simulink model "controller_for_carsim"  (R2021a)
settings: Solver=VariableStepAuto  StartTime=0.0  StopTime=10  RelTol=1e-2
undefined symbols (not defined in the file): Fyf, ks, PredictionHorizon, SlipAngle, Ts, Vx
libraries: mpclib x1, Solver_SF x1, simulink_extras x1, simulink x1
settings Model: Creator=dekunw  LastModifiedBy=chnwa
settings SolverCC: AlgebraicLoopSolver=LineSearch
settings DebuggingCC: SFMachineParentedDataDiag=warning

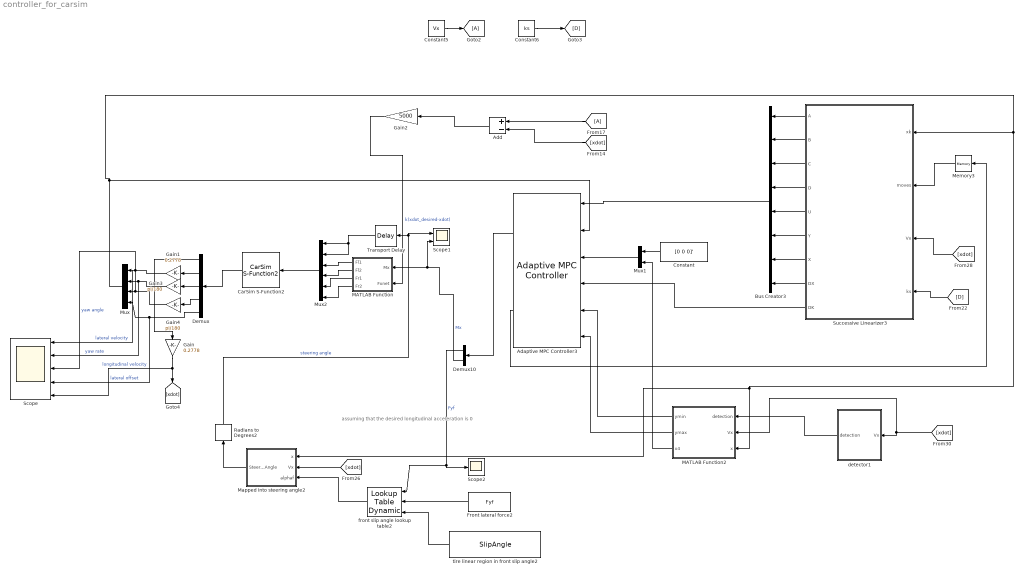
== system controller_for_carsim ==
  note: assuming that the desired longitudinal acceleration is 0
  Adaptive MPC Controller3 : mpclib/Adaptive MPC Controller  SCDEnableBlockLinearizationSpecification=on  mpcobj=mpc007  enable_value=0  updateMPCinCallerWorkspace=on  md_inport=on  mv_inport=off  uref_inport=off  return_cost=off  return_mvseq=on  return_qpstatus=off  return_xseq=off  return_state=off  return_ovseq=off  state_inport=off  isltv_plant=on  umin_inport=off  umax_inport=off  ymin_inport=on  ymax_inport=on  cc_inport=off  ywt_inport=off  uwt_inport=off  duwt_inport=off  rhoeps_inport=off  pm_inport=off  MaximumP=10  HorizonChoice=FixedHorizon  BlockDataType=double  SampleTimeInherited=off  switch_inport=off
  Add : Sum  Inputs=+-
  Bus Creator3 : BusCreator  Inputs=8
  CarSim S-Function2 : Solver_SF/CarSim S-Function2  Priority=1  VehicleCode=i_i  SIMFILE=simfile.sim
      settings: AttributesFormatString=Vehicle Code: %<VehicleCode>
  Constant : Constant  Value=[0 0 0]'
  Constant5 : Constant  Value=Vx
  Constant6 : Constant  Value=ks
  Demux : Demux  Outputs=5
  Demux10 : Demux  Outputs=2
  Front lateral force2 : Constant  Value=Fyf
  Gain : Gain  Gain=0.2778
  Gain1 : Gain  Gain=0.2778
  Gain2 : Gain  Gain=5000
  Gain3 : Gain  Gain=pi/180
  Gain4 : Gain  Gain=pi/180
  MATLAB Function : MATLAB Function  TreatAsAtomicUnit=on
  MATLAB Function2 : MATLAB Function  TreatAsAtomicUnit=on
  Mapped into steering angle2 : MATLAB Function  TreatAsAtomicUnit=on
  Memory3 : Memory
  Mux : Mux
  Mux1 : Mux  Inputs=2
  Mux2 : Mux  Inputs=6
  Radians to Degrees2 : simulink_extras/Transformations/Radians to Degrees
  Scope : Scope  NumInputPorts=5
  Scope1 : Scope  NumInputPorts=2
  Scope2 : Scope
  Successive Linearizer3 : MATLAB Function  TreatAsAtomicUnit=on
  Transport Delay : TransportDelay  DelayTime=Ts
  detector1 : Subsystem
  front slip angle lookup table2 : simulink/Lookup Tables/Lookup Table Dynamic  LookUpMeth=Interpolation-Use End Values  OutDataType=fixdt('double')  OutScaling=[]  OutputDataTypeScalingMode=Specify via dialog  OutDataTypeStr=double  DoSatur=off
  tire linear region in front slip angle2 : Constant  Value=SlipAngle
  wires:
  MATLAB Function2/1(ymin) -> Adaptive MPC Controller3/5
  detector1/1(detection) -> MATLAB Function2/1(detection)
  MATLAB Function2/3(x4) -> Mux1/2
  MATLAB Function2/2(ymax) -> Adaptive MPC Controller3/6
  [xdot] -> MATLAB Function2/2(Vx), detector1/1(Vx)
  Demux10/2 -> Scope1/2, MATLAB Function/1(Mx)  "Mx"
  Successive Linearizer3/9(DK) -> Adaptive MPC Controller3/4
  Successive Linearizer3/4(D) -> Bus Creator3/4
  Mux/1 -> Successive Linearizer3/1(xk), MATLAB Function2/3(x), Mapped into steering angle2/1(x), Adaptive MPC Controller3/2
  tire linear region in front slip angle2/1 -> front slip angle lookup table2/3
  [xdot] -> Mapped into steering angle2/2(Vx)
  Bus Creator3/1 -> Adaptive MPC Controller3/1
  Demux10/1 -> Scope2/1, front slip angle lookup table2/1  "Fyf"
  [xdot] -> Successive Linearizer3/3(Vx)
  Successive Linearizer3/3(C) -> Bus Creator3/3
  Successive Linearizer3/8(DX) -> Bus Creator3/8
  Front lateral force2/1 -> front slip angle lookup table2/2
  Successive Linearizer3/7(X) -> Bus Creator3/7
  Adaptive MPC Controller3/2 -> Memory3/1
  Adaptive MPC Controller3/1 -> Demux10/1
  [xdot] -> Add/2
  [A] -> Add/1
  Add/1 -> Gain2/1
  Transport Delay/1 -> Mux2/2, Mux2/1
  Successive Linearizer3/1(A) -> Bus Creator3/1
  Memory3/1 -> Successive Linearizer3/2(moves)
  Successive Linearizer3/5(U) -> Bus Creator3/5
  [D] -> Successive Linearizer3/4(ks)
  Successive Linearizer3/2(B) -> Bus Creator3/2
  Gain2/1 -> MATLAB Function/2(Fxnet)  "k(xdot_desired-xdot)"
  Radians to Degrees2/1 -> Transport Delay/1, Scope1/1  "steering angle"
  front slip angle lookup table2/1 -> Mapped into steering angle2/3(alphaf)
  Successive Linearizer3/6(Y) -> Bus Creator3/6
  Mapped into steering angle2/1(SteeringAngle) -> Radians to Degrees2/1
  Constant5/1 -> [A]
  Constant6/1 -> [D]
  Demux/1 -> Gain/1
  Gain1/1 -> Scope/1, Mux/1  "lateral velocity"
  Gain3/1 -> Scope/2, Mux/2  "yaw rate"
  Demux/4 -> Gain4/1
  Demux/5 -> Scope/4, Mux/4  "lateral offset"
  Mux2/1 -> CarSim S-Function2/1
  CarSim S-Function2/1 -> Demux/1
  Gain/1 -> [xdot], Scope/5  "longitudinal velocity"
  Demux/2 -> Gain1/1
  Demux/3 -> Gain3/1
  Gain4/1 -> Scope/3, Mux/3  "yaw angle"
  MATLAB Function/1(Fl1) -> Mux2/3
  MATLAB Function/2(Fl2) -> Mux2/4
  MATLAB Function/3(Fr1) -> Mux2/5
  MATLAB Function/4(Fr2) -> Mux2/6
  Mux1/1 -> Adaptive MPC Controller3/3
  Constant/1 -> Mux1/1

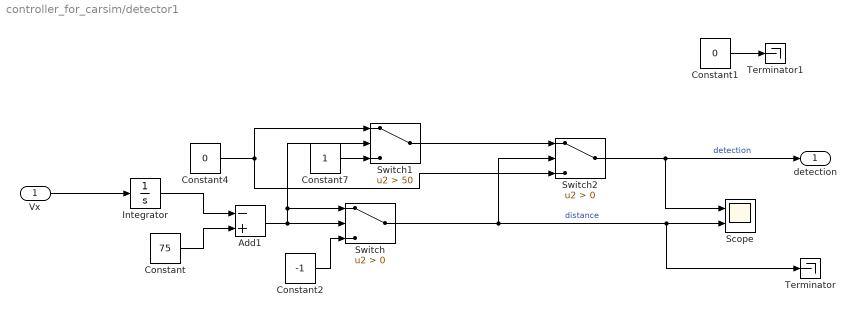
== system controller_for_carsim/detector1 ==
  Vx : Inport
  Add1 : Sum  Inputs=-+
  Constant : Constant  Value=75
  Constant1 : Constant  Value=0
  Constant2 : Constant  Value=-1
  Constant4 : Constant  Value=0
  Constant7 : Constant
  Integrator : Integrator
  Scope : Scope  NumInputPorts=2
  Switch : Switch  Criteria=u2 > Threshold
  Switch1 : Switch  Criteria=u2 > Threshold  Threshold=50
  Switch2 : Switch  Criteria=u2 > Threshold
  Terminator : Terminator
  Terminator1 : Terminator
  detection : Outport
  wires:
  Constant2/1 -> Switch/3
  Constant4/1 -> Switch2/3, Switch1/1
  Vx/1 -> Integrator/1
  Integrator/1 -> Add1/1
  Switch/1 -> Switch2/2, Terminator/1, Scope/2  "distance"
  Constant7/1 -> Switch1/3
  Add1/1 -> Switch1/2, Switch/1, Switch/2
  Switch1/1 -> Switch2/1
  Constant/1 -> Add1/2
  Switch2/1 -> detection/1, Scope/1  "detection"
  Constant1/1 -> Terminator1/1

== matlab function controller_for_carsim/MATLAB Function2 ==
  data: detection input; ymin output; ymax output; Vx input; x input; x4 output
function [ymin,ymax,x4] = fcn(detection,Vx,x)

miu = 0.7; %frction cooeficient 0.7 for dry road and 0.4 for wet
g = 9.81; % gravity
m = 2272;   %mass
lf = 1.11;  % distance from front axle to the mass center
lr = 1.67;  % distance from rear axle to the mass center
C_a = 1.822e5; % rear cornering stifness

Fz = m*g*lf/(lf+lr)/2; % the load that beared by the rear tire

rmax = g*miu/Vx; %max yaw rate
threshold = atan(3*miu*Fz/C_a);

r = x(2);
vmax = lr*r+Vx*threshold;   %max lateral velocity
vmin = lr*r-Vx*threshold;   %min lateral velocity

if detection == 1
    ymin = [vmin -rmax -inf 5]';%50m is the distance from which obstacle is detected
    ymax = [vmax rmax inf 10]';
    x4 = 0;
else
    ymin = [vmin -rmax -pi/2 -10]';
    ymax = [vmax rmax pi/2 10]';
    x4 = 0;
end

== matlab function controller_for_carsim/Mapped into steering angle2 ==
  data: x input; Vx input; alphaf input; SteeringAngle output
function SteeringAngle = fcn(x,Vx, alphaf)

lf = 1.11;  % distance from front axle to the mass center

Vy = x(1); %lateral velocity
r = x(2);  %yaw rate
SteeringAngle = Vy/Vx+lf*r/Vx-alphaf;

== matlab function controller_for_carsim/Successive Linearizer3 ==
  data: A output size=[4,4,PredictionHorizon+1]; xk input size=[4,1]; moves input; B output size=[4,6,PredictionHorizon+1]; C output size=[4,4,PredictionHorizon+1]; D output size=[4,6,PredictionHorizon+1]; U output size=[6,1,PredictionHorizon+1]; Y output size=[4,1,PredictionHorizon+1]; X output size=[4,1,PredictionHorizon+1]; DX output size=[4,1,PredictionHorizon+1]; Vx input size=1; ks input; PredictionHorizon parameter size=1; DK output; Ts parameter size=1
function [A,B,C,D,U,Y,X,DX,DK] = fcn(xk,moves,Vx,ks, PredictionHorizon, Ts)
%sucessive updates the LTI plant model required by adaptive MPC controller

% LTV MPC requires p+1 linearizations from k to k+p
Steps = PredictionHorizon + 1; % having the number of Steps models
% Initialize outputs
A = zeros(4,4,Steps);
B = zeros(4,6,Steps);
C = zeros(4,4,Steps);
D = zeros(4,6,Steps);
U = zeros(6,1,Steps);
Y = zeros(4,1,Steps);
X = zeros(4,1,Steps);
DX = zeros(4,1,Steps);
DK = zeros(Steps,4); % the constant matrix in the model considered as measured disturbance

% Obtain time varying linear models via successive linearization
for ct = 1:Steps
    % since we don't have u(k) ... u(k+p) at the time of linearization,
    % previous optimal sequence u(k-1) ... u(k+p-1) is used instead.
    if ct>length(moves)
        uk = moves(Steps,:);
    else
        uk = moves(ct,:);
    end
    uk = uk';
    % analytical linearization (continuous time)
    [Ac, Bc, Cc, Dc, dc] = LateralDynamicsCT(Vx,ks,xk); % acquiring new characteristic matrix
    % convert A and B matrices from continuous time to discrete time
    % augmenting the model to be in the form of dotX=A*x+B*u while u=[u;dc]
    Aca = Ac;
    Bca = [Bc eye(4)];
    M = expm([[Aca Bca zeros(4,1)]*Ts;zeros(7,11)]);
    Ak = M(1:4,1:4);    %the discrete matrix A for augmented model
    Bk = M(1:4,5:10);   %the discrete matrix B for augmented model
    %store the state space matrix for ct time step
    A(:,:,ct) = Ak;
    B(:,:,ct) = Bk;
    C(:,:,ct) = Cc;
    D(:,:,ct) = [Dc,zeros(4,4)];  % always be zeros(4,6) in fact
    U(:,:,ct) = [uk;dc];          % measured disturbance dc is input as well
    Y(:,:,ct) = xk;               % output is all of the four states
    X(:,:,ct) = xk;               % four states
    DX(:,:,ct) = Ak*xk+Bk*[uk;dc]-xk;%the states increment
    DK(ct,:) = dc';               % disturbance in this step
    % next prediction step
    xk = DX(:,:,ct)+xk;           %update the states
end

%%%unrelated stuff
% ct= LTVu15_dist_Ts01.Model.Plant;
% dt = c2d(ct,Ts);
% LTVu15_dist_Ts01.Model.Plant = dt;

== matlab function controller_for_carsim/MATLAB Function ==
  data: Fl1 output; Mx input; Fl2 output; Fxnet input; Fr1 output; Fr2 output
function [Fl1,Fl2,Fr1,Fr2] = fcn(Mx,Fxnet)

w = 1.875; % the width of the car

Fwf = zeros(2,1);
Fwr = zeros(2,1);

if Mx > 0
    Fwf(1) = Fxnet/2+0;
    Fwf(2) = Fxnet/2-Mx/w;
    Fwr(1) = 0;
    Fwr(2) = -Mx/w;
elseif Mx < 0
    Fwf(1) = Fxnet/2+Mx/w;
    Fwf(2) = Fxnet/2+0;
    Fwr(1) = Mx/w;
    Fwr(2) = 0;
else
    Fwf(1) = Fxnet/2+0;
    Fwf(2) = Fxnet/2+0;
    Fwr(1) = 0;
    Fwr(2) = 0;
end
Fl1 = Fwf(1);
Fl2 = Fwr(1);
Fr1 = Fwf(2);
Fr2 = Fwr(2);
